simulink model "prob_10"  (R2020b)
settings: Solver=VariableStepAuto  StartTime=0.0  StopTime=10.0  RelTol=1e-3
settings Model: Creator=Akshay A H  LastModifiedBy=Akshay A H

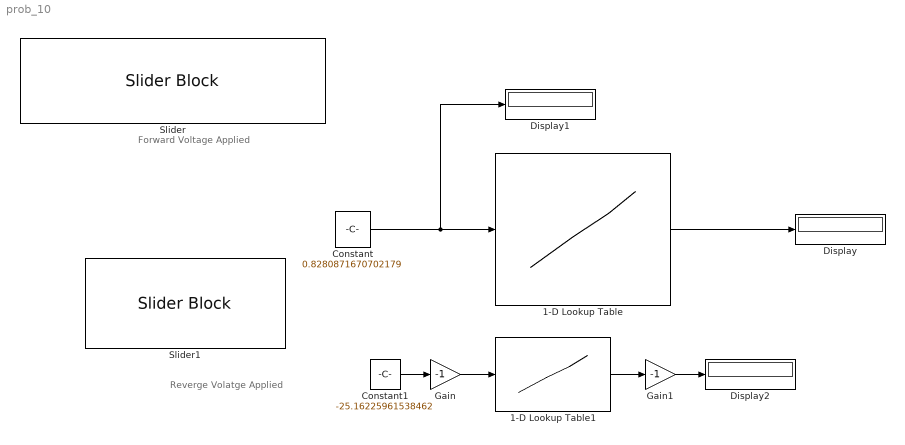
== system prob_10 ==
  note: Reverge Volatge Applied
  note: Forward Voltage Applied
  1-D Lookup Table : Lookup_n-D  NumberOfTableDimensions=1  BreakpointsForDimension1=[0.12,0.14,0.16,0.18,0.20,0.24,0.26,0.28,0.30,0.35,0.38,0.40]  BreakpointsForDimension2=[-150,-100,-50]  Table=[0.01,0.02,0.03,0.04,0.05,0.06,0.08,0.12,0.20,0.25,5,10]  InternalRulePriority=Speed  RndMeth=Simplest  InputSameDT=on
  1-D Lookup Table1 : Lookup_n-D  NumberOfTableDimensions=1  BreakpointsForDimension1=[0.5,1,10,14,14.5,14.7]  Table=[5,5,5,5,200,400]  InternalRulePriority=Speed  RndMeth=Simplest  InputSameDT=on
  Constant : Constant  Value=0.8280871670702179
  Constant1 : Constant  Value=-25.16225961538462
  Display : Display
  Display1 : Display
  Display2 : Display
  Gain : Gain  Gain=-1
  Gain1 : Gain  Gain=-1
  Slider : SliderBlock  ScaleMax=3
  Slider1 : SliderBlock  ScaleMin=-50  ScaleMax=0
  wires:
  Constant1/1 -> Gain/1
  Gain/1 -> 1-D Lookup Table1/1
  1-D Lookup Table/1 -> Display/1
  1-D Lookup Table1/1 -> Gain1/1
  Constant/1 -> Display1/1, 1-D Lookup Table/1
  Gain1/1 -> Display2/1
